simulink model "clean_SU"  (R2021a)
settings: Solver=VariableStepAuto  StartTime=0.0  StopTime=stop  FixedStep=0.005  MaxStep=maxdt  MinStep=maxdt/100  RelTol=1e-5
values from neighbouring files (symbols this model uses):
  a_1M = Mu1/J1K    (= 0.0028830906732)    [NASTROYKI.m]    (also in NASTROYKI_STAB.m; NASTROYKI_VSEGO.m)
  a_2M = Mu2/J2K    (= 0.00292525961679)    [NASTROYKI.m]    (also in NASTROYKI_STAB.m; NASTROYKI_VSEGO.m)
  a_3M = Mu3/J3K    (= 0.017825311943)    [NASTROYKI.m]    (also in NASTROYKI_STAB.m; NASTROYKI_VSEGO.m)
  alpha_1M = 0.9*Xmax1    (= 27)    [NASTROYKI.m]    (also in NASTROYKI_STAB.m; NASTROYKI_VSEGO.m)
  alpha_2M = 0.9*Xmax2    (= 27)    [NASTROYKI.m]    (also in NASTROYKI_STAB.m; NASTROYKI_VSEGO.m)
  alpha_3M = 0.9*Xmax3    (= 27)    [NASTROYKI.m]    (also in NASTROYKI_STAB.m; NASTROYKI_VSEGO.m)
  DtR = pi/180    (= 0.0174532925199)    [NASTROYKI.m]    (also in NASTROYKI_STAB.m; NASTROYKI_VSEGO.m)
  g_1M = g_1M+MuR/J1K    (= 3.60530488684e-06)    [NASTROYKI.m]    (also in NASTROYKI_STAB.m; NASTROYKI_VSEGO.m = 7.20916822834e-06)
  g_2M = g_2M+MuR/J2K    (= 3.65672078397e-06)    [NASTROYKI.m]    (also in NASTROYKI_STAB.m; NASTROYKI_VSEGO.m = 7.31329530496e-06)
  g_3M = g_3M+MuR/J3K    (= 2.22905525847e-05)    [NASTROYKI.m]    (also in NASTROYKI_STAB.m; NASTROYKI_VSEGO.m = 4.45721925134e-05)
  h_1M = 0.2*alpha_1M    (= 5.4)    [NASTROYKI.m]    (also in NASTROYKI_STAB.m; NASTROYKI_VSEGO.m)
  h_2M = 0.2*alpha_2M    (= 5.4)    [NASTROYKI.m]    (also in NASTROYKI_STAB.m; NASTROYKI_VSEGO.m)
  h_3M = 0.2*alpha_3M    (= 5.4)    [NASTROYKI.m]    (also in NASTROYKI_STAB.m; NASTROYKI_VSEGO.m)
  J1K = 6937    [NASTROYKI.m]    (also in NASTROYKI_STAB.m; NASTROYKI_VSEGO.m)
  J1M = 2    [NASTROYKI.m]    (also in NASTROYKI_STAB.m; NASTROYKI_VSEGO.m)
  J2K = 6837    [NASTROYKI.m]    (also in NASTROYKI_STAB.m; NASTROYKI_VSEGO.m)
  J2M = 2    [NASTROYKI.m]    (also in NASTROYKI_STAB.m; NASTROYKI_VSEGO.m)
  J3K = 1122    [NASTROYKI.m]    (also in NASTROYKI_STAB.m; NASTROYKI_VSEGO.m)
  J3M = 2    [NASTROYKI.m]    (also in NASTROYKI_STAB.m; NASTROYKI_VSEGO.m)
  k_1M = h_1M/(2*yZV)    (= 2.7)    [NASTROYKI.m]    (also in NASTROYKI_STAB.m; NASTROYKI_VSEGO.m)
  k_2M = h_2M/(2*yZV)    (= 2.7)    [NASTROYKI.m]    (also in NASTROYKI_STAB.m; NASTROYKI_VSEGO.m)
  k_3M = h_3M/(2*yZV)    (= 2.7)    [NASTROYKI.m]    (also in NASTROYKI_STAB.m; NASTROYKI_VSEGO.m)
  L03 = 0    [NASTROYKI.m]    (also in NASTROYKI_STAB.m; NASTROYKI_VSEGO.m = 10)
  refT = 5    [NASTROYKI.m]    (also in NASTROYKI_VSEGO.m = 0.1)
  RtD = 1/DtR    (= 57.2957795131)    [NASTROYKI.m]    (also in NASTROYKI_STAB.m; NASTROYKI_VSEGO.m)
  x_0_1M = xZV    (= 30)    [NASTROYKI.m]    (also in NASTROYKI_STAB.m; NASTROYKI_VSEGO.m)
  x_0_2M = xZV    (= 30)    [NASTROYKI.m]    (also in NASTROYKI_STAB.m; NASTROYKI_VSEGO.m)
  x_0_3M = xZV    (= 30)    [NASTROYKI.m]    (also in NASTROYKI_STAB.m; NASTROYKI_VSEGO.m)
  y_0_1M = yZV    (= 1)    [NASTROYKI.m]    (also in NASTROYKI_STAB.m; NASTROYKI_VSEGO.m)
  y_0_2M = yZV    (= 1)    [NASTROYKI.m]    (also in NASTROYKI_STAB.m; NASTROYKI_VSEGO.m)
  y_0_3M = yZV    (= 1)    [NASTROYKI.m]    (also in NASTROYKI_STAB.m; NASTROYKI_VSEGO.m)
undefined symbols (not defined in the file or in its folder): Earth, WGS84
libraries: aerolibanim x4, templibrary x3, aerolibfltsims x2, aerolibtransform2 x1
settings Model: SimulationMode=rapid-accelerator  Creator=vanya  LastModifiedBy=vanya
settings SolverCC: ZeroCrossControl=DisableAll

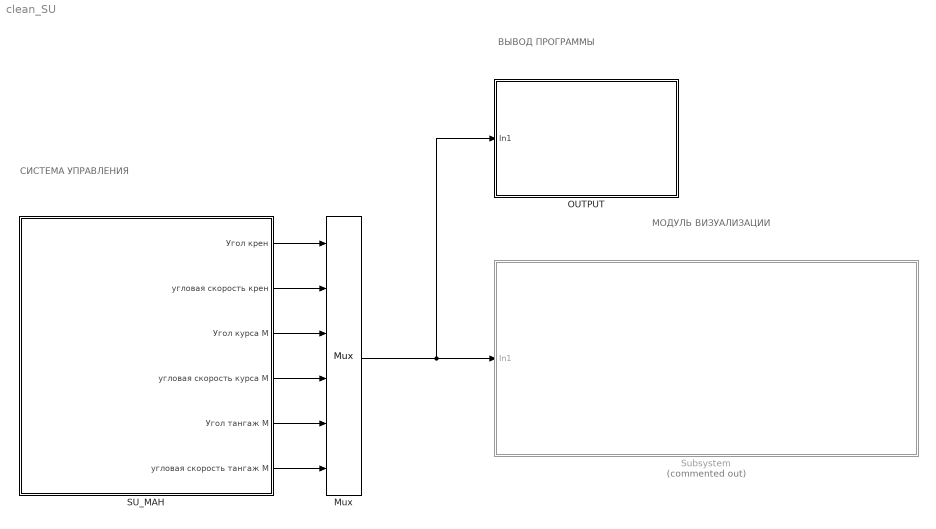
== system clean_SU ==
  note: МОДУЛЬ ВИЗУАЛИЗАЦИИ
  note: ВЫВОД ПРОГРАММЫ
  note: СИСТЕМА УПРАВЛЕНИЯ
  Mux : Mux  Inputs=6
  OUTPUT : Subsystem
  SU_MAH : Subsystem
  Subsystem : Subsystem  Commented=on
  wires:
  SU_MAH/1(Угол крен) -> Mux/1
  SU_MAH/2(угловая скорость крен) -> Mux/2
  SU_MAH/3(Угол курса М) -> Mux/3
  SU_MAH/4(угловая скорость курса М) -> Mux/4
  SU_MAH/5(Угол тангаж М) -> Mux/5
  SU_MAH/6(угловая скорость тангаж М) -> Mux/6
  Mux/1 -> OUTPUT/1(In1), Subsystem/1(In1)

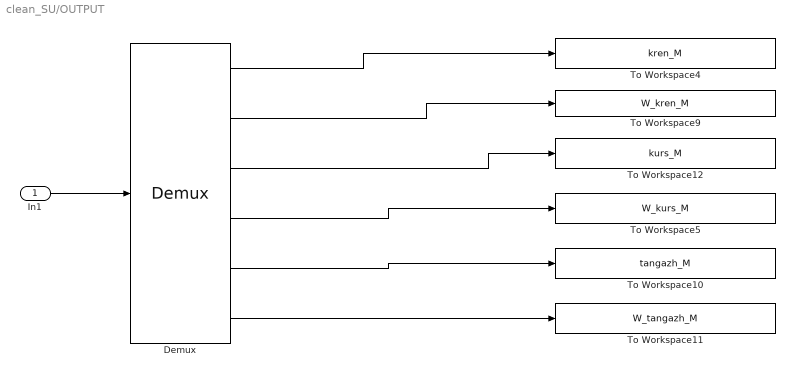
== system clean_SU/OUTPUT ==
  In1 : Inport
  Demux : Demux  Outputs=6
  To Workspace10 : ToWorkspace  VariableName=tangazh_M  SampleTime=-1
      settings: Save2DSignal=2-D array (concatenate along first dimension)
  To Workspace11 : ToWorkspace  VariableName=W_tangazh_M  SampleTime=-1
      settings: Save2DSignal=2-D array (concatenate along first dimension)
  To Workspace12 : ToWorkspace  VariableName=kurs_M  SampleTime=-1
      settings: Save2DSignal=2-D array (concatenate along first dimension)
  To Workspace4 : ToWorkspace  VariableName=kren_M  SampleTime=-1
      settings: Save2DSignal=2-D array (concatenate along first dimension)
  To Workspace5 : ToWorkspace  VariableName=W_kurs_M  SampleTime=-1
      settings: Save2DSignal=2-D array (concatenate along first dimension)
  To Workspace9 : ToWorkspace  VariableName=W_kren_M  SampleTime=-1
      settings: Save2DSignal=2-D array (concatenate along first dimension)
  wires:
  Demux/3 -> To Workspace12/1
  Demux/2 -> To Workspace9/1
  Demux/4 -> To Workspace5/1
  Demux/6 -> To Workspace11/1
  Demux/1 -> To Workspace4/1
  Demux/5 -> To Workspace10/1
  In1/1 -> Demux/1

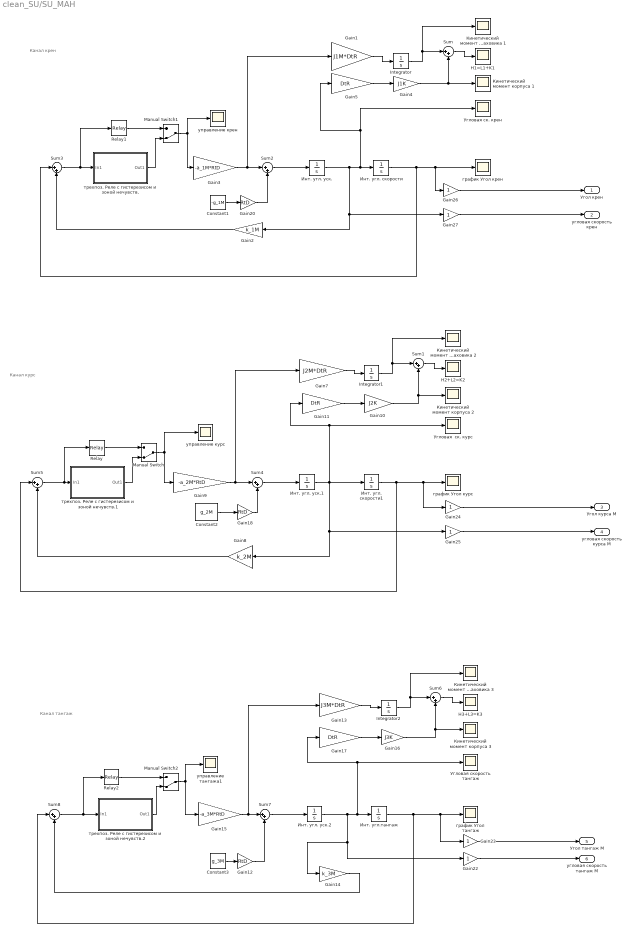
== system clean_SU/SU_MAH ==
  note: Канал
      | крен
  note: Канал
      | курс
  note: Канал
      | тангаж
  " Кинетический момент корпуса 1" : Scope
  " Кинетический момент корпуса 2" : Scope
  " Кинетический момент корпуса 3" : Scope
  Constant1 : Constant  Value=-g_1M
  Constant2 : Constant  Value=g_2M
  Constant3 : Constant  Value=g_3M
  Gain1 : Gain  Gain=J1M*DtR
  Gain10 : Gain  Gain=J2K
  Gain11 : Gain  Gain=DtR
  Gain12 : Gain  Gain=RtD
  Gain13 : Gain  Gain=J3M*DtR
  Gain14 : Gain  Gain=k_3M
  Gain15 : Gain  Gain=-a_3M*RtD
  Gain16 : Gain  Gain=J3K
  Gain17 : Gain  Gain=DtR
  Gain18 : Gain  Gain=RtD
  Gain2 : Gain  Gain=k_1M
  Gain20 : Gain  Gain=RtD
  Gain{22..27} (6 alike) : Gain
  Gain3 : Gain  Gain=-a_1M*RtD
  Gain4 : Gain  Gain=J1K
  Gain5 : Gain  Gain=DtR
  Gain7 : Gain  Gain=J2M*DtR
  Gain8 : Gain  Gain=k_2M
  Gain9 : Gain  Gain=-a_2M*RtD
  H1=L1+K1 : Scope
  H2+L2=K2 : Scope
  H3+L3=K3 : Scope
  Integrator : Integrator
  Integrator1 : Integrator
  Integrator2 : Integrator  InitialCondition=L03
  Manual Switch : ManualSwitch  CurrentSetting=0
  Manual Switch1 : ManualSwitch  CurrentSetting=0
  Manual Switch2 : ManualSwitch  CurrentSetting=0
  Relay : Relay  OnSwitchValue=0  OffSwitchValue=0  OffOutputValue=-1
  Relay1 : Relay  OnSwitchValue=0  OffSwitchValue=0  OffOutputValue=-1
  Relay2 : Relay  OnSwitchValue=0  OffSwitchValue=0  OffOutputValue=-1
  Sum{,1..8} (9 alike) : Sum  Inputs=|++
  Инт. угл. скорости : Integrator  InitialCondition=x_0_1M
  Инт. угл. скорости1 : Integrator  InitialCondition=x_0_2M
  Инт. угл. уск. : Integrator  InitialCondition=y_0_1M
  Инт. угл. уск.1 : Integrator  InitialCondition=y_0_2M
  Инт. угл. уск.2 : Integrator  InitialCondition=y_0_3M
  Инт. угл.тангаж : Integrator  InitialCondition=x_0_3M
  Кинетический момент маховика 1 : Scope
  Кинетический момент маховика 2 : Scope
  Кинетический момент маховика 3 : Scope
  Угловая  ск. курс : Scope
  Угловая ск. крен : Scope
  Угловая скорость тангаж : Scope
  график Угол крен : Scope
  график Угол курс : Scope
  график Угол тангаж : Scope
  трехпоз. Реле с гистерезисом и зоной нечувств. : Subsystem
  трехпоз. Реле с гистерезисом и зоной нечувств.1 : Subsystem
  трехпоз. Реле с гистерезисом и зоной нечувств.2 : Subsystem
  управление крен : Scope
  управление курс : Scope
  управление тангажа1 : Scope
  Угол крен : Outport
  угловая скорость крен : Outport  Port=2
  Угол курса М : Outport  Port=3
  угловая скорость курса М : Outport  Port=4
  Угол тангаж М : Outport  Port=5
  угловая скорость тангаж М : Outport  Port=6
  wires:
  Gain27/1 -> угловая скорость крен/1
  Gain16/1 -> " Кинетический момент корпуса 3"/1, Sum6/2
  Gain25/1 -> угловая скорость курса М/1
  Gain9/1 -> Gain7/1, Sum4/1
  Integrator2/1 -> Кинетический момент маховика 3/1, Sum6/1
  Gain2/1 -> Sum3/2
  Инт. угл.тангаж/1 -> график Угол тангаж/1, Gain23/1, Sum8/1
  Gain22/1 -> угловая скорость тангаж М/1
  Gain26/1 -> Угол крен/1
  Gain24/1 -> Угол курса М/1
  Инт. угл. скорости/1 -> Gain26/1, график Угол крен/1, Sum3/1
  Gain23/1 -> Угол тангаж М/1
  Инт. угл. уск.1/1 -> Инт. угл. скорости1/1, Угловая  ск. курс/1, Gain11/1, Gain25/1, Gain8/1
  Sum6/1 -> H3+L3=K3/1
  Sum/1 -> H1=L1+K1/1
  Инт. угл. уск.2/1 -> Gain22/1, Gain14/1, Угловая скорость тангаж/1, Gain17/1, Инт. угл.тангаж/1
  Gain10/1 -> " Кинетический момент корпуса 2"/1, Sum1/2
  Sum2/1 -> Инт. угл. уск./1
  Gain15/1 -> Gain13/1, Sum7/1
  Gain14/1 -> Sum8/2
  Gain13/1 -> Integrator2/1
  Integrator/1 -> Кинетический момент маховика 1/1, Sum/1
  Gain17/1 -> Gain16/1
  Инт. угл. скорости1/1 -> график Угол курс/1, Gain24/1, Sum5/1
  Gain5/1 -> Gain4/1
  Integrator1/1 -> Кинетический момент маховика 2/1, Sum1/1
  Sum8/1 -> трехпоз. Реле с гистерезисом и зоной нечувств.2/1(In1), Relay2/1
  Инт. угл. уск./1 -> Gain27/1, Gain2/1, Gain5/1, Угловая ск. крен/1, Инт. угл. скорости/1
  Gain3/1 -> Gain1/1, Sum2/1
  Gain11/1 -> Gain10/1
  Sum3/1 -> трехпоз. Реле с гистерезисом и зоной нечувств./1(In1), Relay1/1
  Sum4/1 -> Инт. угл. уск.1/1
  Gain8/1 -> Sum5/2
  Gain7/1 -> Integrator1/1
  Sum1/1 -> H2+L2=K2/1
  Gain1/1 -> Integrator/1
  Gain4/1 -> " Кинетический момент корпуса 1"/1, Sum/2
  Sum7/1 -> Инт. угл. уск.2/1
  Constant3/1 -> Gain12/1
  Gain12/1 -> Sum7/2
  Constant2/1 -> Gain18/1
  Gain18/1 -> Sum4/2
  Constant1/1 -> Gain20/1
  Gain20/1 -> Sum2/2
  трехпоз. Реле с гистерезисом и зоной нечувств.1/1(Out1) -> Manual Switch/2
  Manual Switch/1 -> управление курс/1, Gain9/1
  Sum5/1 -> Relay/1, трехпоз. Реле с гистерезисом и зоной нечувств.1/1(In1)
  Relay/1 -> Manual Switch/1
  Relay1/1 -> Manual Switch1/1
  трехпоз. Реле с гистерезисом и зоной нечувств./1(Out1) -> Manual Switch1/2
  Manual Switch1/1 -> Gain3/1, управление крен/1
  Relay2/1 -> Manual Switch2/1
  Manual Switch2/1 -> Gain15/1, управление тангажа1/1
  трехпоз. Реле с гистерезисом и зоной нечувств.2/1(Out1) -> Manual Switch2/2

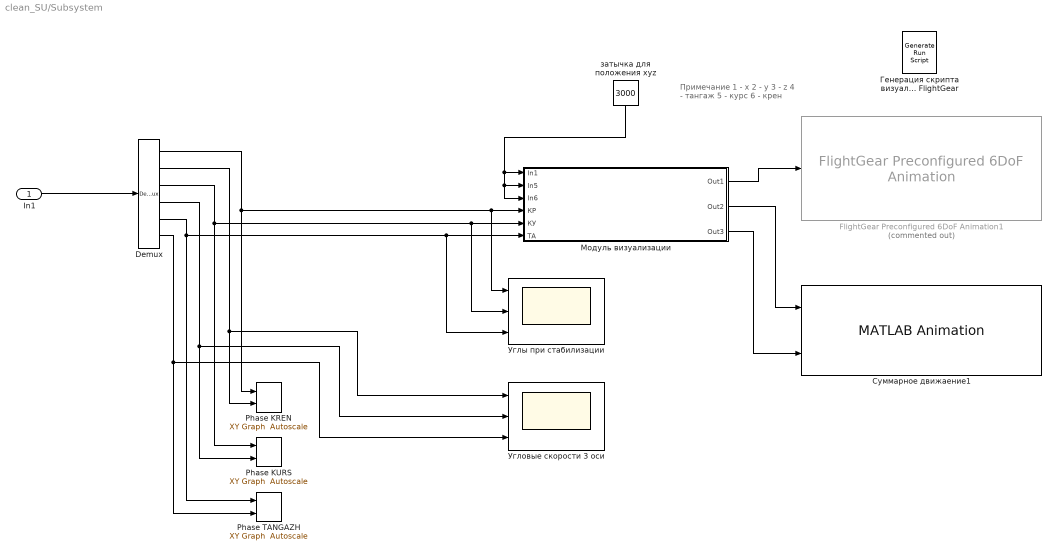
== system clean_SU/Subsystem ==
  note: Примечание
      | 1 - x
      | 2 - y
      | 3 - z
      | 4 - тангаж
      | 5 - курс
      | 6 - крен
  In1 : Inport
  Demux : Demux  Outputs=6
  FlightGear Preconfigured 6DoF Animation1 : aerolibfltsims/FlightGear Preconfigured 6DoF Animation  Commented=on  xFlightGearVersion=v2017.3  DestinationIpAddress=127.0.0.1  DestinationPort=5502  SampleTime=1  packetVersion=24
  Phase KREN : templibrary/XY Graph  Autoscale  xmin=-1  xmax=1  ymin=-1  ymax=1  st=-1
  Phase KURS : templibrary/XY Graph  Autoscale  xmin=-1  xmax=1  ymin=-1  ymax=1  st=-1
  Phase TANGAZH : templibrary/XY Graph  Autoscale  xmin=-1  xmax=1  ymin=-1  ymax=1  st=-1
  Генерация скрипта визуализации в FlightGear : aerolibfltsims/Generate Run Script  Architecture=Default  dataFlow=Send  GeometryModelName=14bis  AirportId=KSFO  RunwayId=10L  InitialAltitude=722*100  InitialHeading=113  OffsetDistance=4.72  OffsetAzimuth=0  InstallScenery=off  DisableShaders=off  OriginAddress=127.0.0.1  DestinationPort=5502  OriginPort=5505  LocalAddress=127.0.0.1  OutputFileName=runfg.bat  FlightGearBaseDirectory=C:\Program Files\FlightGear 2020.3
  Модуль визуализации : Subsystem
  Суммарное движаение1 : aerolibanim/MATLAB Animation  Tag=Matlab Animation 6 DOF  Vehicles=1  Geometries=Geometry  BoundingBoxCoordinates=[-50,50,-50,50,-50,50]  CameraOffset=[150,-150,-150]  CameraViewAngle=1  SampleTime=refT  FigurePosition=[1019,170,741,507]
      settings: SourceProductBaseCode=AE
  Угловые скорости 3 оси : Scope  NumInputPorts=3
  Углы при стабилизации : Scope  NumInputPorts=3
  затычка для положения xyz : Constant  Value=3000
  wires:
  Модуль визуализации/3(Out3) -> Суммарное движаение1/2
  затычка для положения xyz/1 -> Модуль визуализации/1(In1), Модуль визуализации/3(In6), Модуль визуализации/2(In5)
  Модуль визуализации/2(Out2) -> Суммарное движаение1/1
  Модуль визуализации/1(Out1) -> FlightGear Preconfigured 6DoF Animation1/1
  Demux/2 -> Phase KREN/2, Угловые скорости 3 оси/1
  Demux/4 -> Phase KURS/2, Угловые скорости 3 оси/2
  Demux/6 -> Phase TANGAZH/2, Угловые скорости 3 оси/3
  Demux/1 -> Углы при стабилизации/1, Модуль визуализации/4(КР), Phase KREN/1
  Demux/3 -> Модуль визуализации/5(КУ), Углы при стабилизации/2, Phase KURS/1
  In1/1 -> Demux/1
  Demux/5 -> Phase TANGAZH/1, Углы при стабилизации/3, Модуль визуализации/6(ТА)

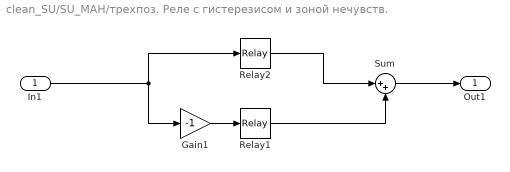
== system clean_SU/SU_MAH/трехпоз. Реле с гистерезисом и зоной нечувств. ==
  In1 : Inport
  Gain1 : Gain  Gain=-1
  Relay1 : Relay  OnSwitchValue=alpha_1M  OffSwitchValue=alpha_1M-h_1M  OnOutputValue=-1
  Relay2 : Relay  OnSwitchValue=alpha_1M  OffSwitchValue=alpha_1M-h_1M
  Sum : Sum  Inputs=|++
  Out1 : Outport
  wires:
  Gain1/1 -> Relay1/1
  In1/1 -> Gain1/1, Relay2/1
  Sum/1 -> Out1/1
  Relay1/1 -> Sum/2
  Relay2/1 -> Sum/1

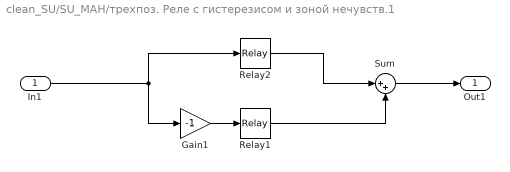
== system clean_SU/SU_MAH/трехпоз. Реле с гистерезисом и зоной нечувств.1 ==
  In1 : Inport
  Gain1 : Gain  Gain=-1
  Relay1 : Relay  OnSwitchValue=alpha_2M  OffSwitchValue=alpha_2M-h_2M  OnOutputValue=-1
  Relay2 : Relay  OnSwitchValue=alpha_2M  OffSwitchValue=alpha_2M-h_2M
  Sum : Sum  Inputs=|++
  Out1 : Outport
  wires:
  Gain1/1 -> Relay1/1
  In1/1 -> Gain1/1, Relay2/1
  Sum/1 -> Out1/1
  Relay1/1 -> Sum/2
  Relay2/1 -> Sum/1

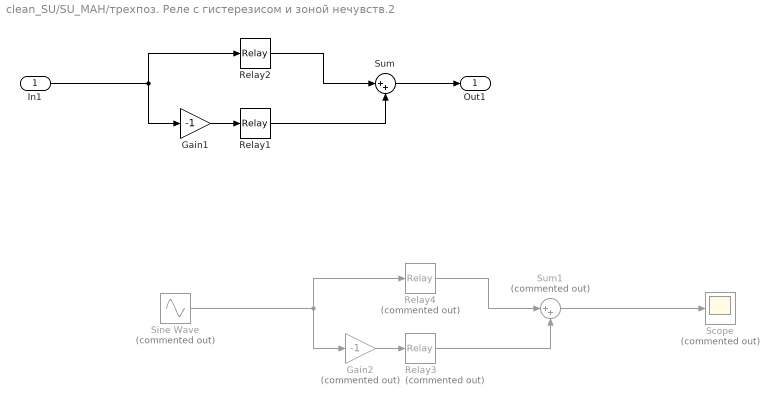
== system clean_SU/SU_MAH/трехпоз. Реле с гистерезисом и зоной нечувств.2 ==
  In1 : Inport
  Gain1 : Gain  Gain=-1
  Gain2 : Gain  Commented=on  Gain=-1
  Relay1 : Relay  OnSwitchValue=alpha_3M  OffSwitchValue=alpha_3M-h_3M  OnOutputValue=-1
  Relay2 : Relay  OnSwitchValue=alpha_3M  OffSwitchValue=alpha_3M-h_3M
  Relay3 : Relay  Commented=on  OnSwitchValue=1  OffSwitchValue=0.5  OnOutputValue=-1
  Relay4 : Relay  Commented=on  OnSwitchValue=1  OffSwitchValue=0.5
  Scope : Scope  Commented=on
  Sine Wave : Sin  Commented=on  Amplitude=2  SampleTime=0
  Sum : Sum  Inputs=|++
  Sum1 : Sum  Commented=on  Inputs=|++
  Out1 : Outport
  wires:
  Gain1/1 -> Relay1/1
  In1/1 -> Gain1/1, Relay2/1
  Sum/1 -> Out1/1
  Relay1/1 -> Sum/2
  Relay2/1 -> Sum/1
  Relay4/1 -> Sum1/1
  Relay3/1 -> Sum1/2
  Sine Wave/1 -> Gain2/1, Relay4/1
  Gain2/1 -> Relay3/1
  Sum1/1 -> Scope/1

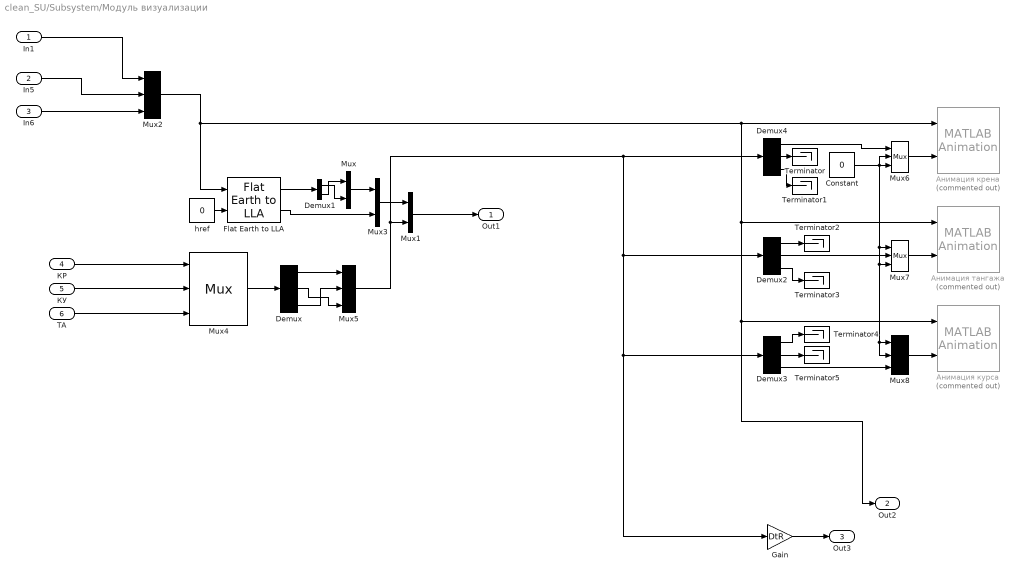
== system clean_SU/Subsystem/Модуль визуализации ==
  In1 : Inport
  In5 : Inport  Port=2
  In6 : Inport  Port=3
  КР : Inport  Port=4
  КУ : Inport  Port=5
  ТА : Inport  Port=6
  Constant : Constant  Value=0
  Demux{,2..4} (4 alike) : Demux  Outputs=3
  Demux1 : Demux  Outputs=2
  Flat Earth to LLA : aerolibtransform2/Flat Earth to LLA  units=Metric (MKS)  ptype=Earth (WGS84)  F=1/298.257223563  R=6378137  refPosPort=off  LL0=[37.61 -122.39]  psi=0
  Gain : Gain  Gain=DtR
  Mux : Mux  Inputs=2
  Mux1 : Mux  Inputs=2
  Mux{2,4..8} (6 alike) : Mux  Inputs=3
  Mux3 : Mux  Inputs=2
  Terminator{,1..5} (6 alike) : Terminator
  href : Constant  Value=0
  Анимация крена : aerolibanim/MATLAB Animation  Tag=Matlab Animation 6 DOF  Commented=on  Vehicles=1  Geometries='astredwedge.mat'  BoundingBoxCoordinates=[-50,50,-50,50,-50,50]  CameraOffset=[-50,-50,-50]  CameraViewAngle=2  SampleTime=0.2  FigurePosition=[786,232,729,287]
      settings: SourceProductBaseCode=AE
  Анимация курса : aerolibanim/MATLAB Animation  Tag=Matlab Animation 6 DOF  Commented=on  Vehicles=1  Geometries='astredwedge.mat'  BoundingBoxCoordinates=[-50,50,-50,50,-50,50]  CameraOffset=[0,0,-400]  CameraViewAngle=1  SampleTime=0.2  FigurePosition=[529,247,612,404]
      settings: SourceProductBaseCode=AE
  Анимация тангажа : aerolibanim/MATLAB Animation  Tag=Matlab Animation 6 DOF  Commented=on  Vehicles=1  Geometries='astredwedge.mat'  BoundingBoxCoordinates=[-50,50,-50,50,-50,50]  CameraOffset=[-50,-50,-50]  CameraViewAngle=2  SampleTime=0.2  FigurePosition=[447,306,729,287]
      settings: SourceProductBaseCode=AE
  Out1 : Outport
  Out2 : Outport  Port=2
  Out3 : Outport  Port=3
  wires:
  Demux1/2 -> Mux/1
  Mux4/1 -> Demux/1
  Flat Earth to LLA/1 -> Demux1/1
  Mux/1 -> Mux3/1
  Mux3/1 -> Mux1/1
  href/1 -> Flat Earth to LLA/2
  Flat Earth to LLA/2 -> Mux3/2
  Mux1/1 -> Out1/1
  Demux1/1 -> Mux/2
  In1/1 -> Mux2/1
  In5/1 -> Mux2/2
  In6/1 -> Mux2/3
  Demux4/3 -> Terminator1/1
  Demux3/1 -> Terminator4/1
  Mux7/1 -> Анимация тангажа/2
  Demux3/2 -> Terminator5/1
  Demux2/1 -> Terminator2/1
  Demux2/2 -> Mux7/2
  Mux6/1 -> Анимация крена/2
  Demux3/3 -> Mux8/3
  Demux4/2 -> Terminator/1
  Constant/1 -> Mux7/3, Mux8/2, Mux8/1, Mux7/1, Mux6/2, Mux6/3
  Demux4/1 -> Mux6/1
  Mux8/1 -> Анимация курса/2
  Demux2/3 -> Terminator3/1
  Mux2/1 -> Анимация крена/1, Анимация тангажа/1, Анимация курса/1, Out2/1, Flat Earth to LLA/1
  Mux5/1 -> Demux4/1, Demux2/1, Gain/1, Demux3/1, Mux1/2
  КР/1 -> Mux4/1
  КУ/1 -> Mux4/2
  ТА/1 -> Mux4/3
  Demux/1 -> Mux5/1
  Demux/3 -> Mux5/2
  Demux/2 -> Mux5/3
  Gain/1 -> Out3/1
